simulink model "untitled"  (R2016b)
settings: Solver=VariableStepAuto  StartTime=0.0  StopTime=10.0  RelTol=1e-3
undefined symbols (not defined in the file): K, Kp, w0, z
settings Model: Creator=emiliendurif  LastModifiedBy=emiliendurif

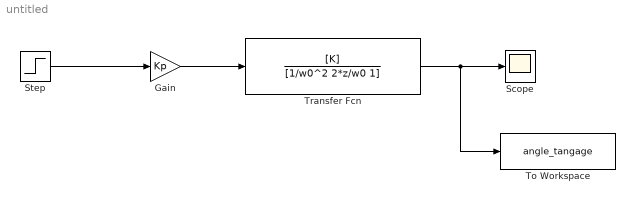
== system untitled ==
  Gain : Gain  Gain=Kp
  Scope : Scope
  Step : Step  SampleTime=0
  To Workspace : ToWorkspace  VariableName=angle_tangage  SaveFormat=Timeseries  SampleTime=-1
  Transfer Fcn : TransferFcn  Numerator=[K]  Denominator=[1/w0^2 2*z/w0 1]
  wires:
  Transfer Fcn/1 -> To Workspace/1, Scope/1
  Gain/1 -> Transfer Fcn/1
  Step/1 -> Gain/1
